simulink model "APP_ChkSig1"  (R2016b)
settings: configuration reference "CodeGenConfigSet" (kept outside this file)
values from neighbouring files (symbols this model uses):
  APP_drLimNeg_C = Calibration.Parameter    [init_APP_ChkSig.m]    (also in init_APP_ChkSig_SIL.m = Simulink.Parameter)
  APP_drLimpMax_C = Calibration.Parameter    [init_APP_ChkSig.m]    (also in init_APP_ChkSig_SIL.m = Simulink.Parameter)
  APP_drLimPos_C = Calibration.Parameter    [init_APP_ChkSig.m]    (also in init_APP_ChkSig_SIL.m = Simulink.Parameter)
  APP_rLimpMax_C = Calibration.Parameter    [init_APP_ChkSig.m]    (also in init_APP_ChkSig_SIL.m = Simulink.Parameter)
  APP_rPlaMaxVal_C = Calibration.Parameter    [init_APP_ChkSig.m]    (also in init_APP_ChkSig_SIL.m = Simulink.Parameter)
  APP_rRmtAPPThresTrqDem_C = Calibration.Parameter    [init_APP_ChkSig.m]    (also in init_APP_ChkSig_SIL.m = Simulink.Parameter)
  APP_rRmtAPPThresTrqDemH_C = Calibration.Parameter    [init_APP_ChkSig.m]    (also in init_APP_ChkSig_SIL.m = Simulink.Parameter)
  APP_rRmtAPPThresTrqDemL_C = Calibration.Parameter    [init_APP_ChkSig.m]    (also in init_APP_ChkSig_SIL.m = Simulink.Parameter)
  APP_rThresAliveDet_C = Calibration.Parameter    [init_APP_ChkSig.m]    (also in init_APP_ChkSig_SIL.m = Simulink.Parameter)
  APP_stRmtAppTrqEN_C = Calibration.Parameter    [init_APP_ChkSig.m]    (also in init_APP_ChkSig_SIL.m = Simulink.Parameter)
  APP_swtAliveDetEna_C = Calibration.Parameter    [init_APP_ChkSig.m]    (also in init_APP_ChkSig_SIL.m = Simulink.Parameter)
  APP_swtPlaChkEna_C = Calibration.Parameter    [init_APP_ChkSig.m]    (also in init_APP_ChkSig_SIL.m = Simulink.Parameter)
  APP_tiAliveDebHiLo_C = Calibration.Parameter    [init_APP_ChkSig.m]    (also in init_APP_ChkSig_SIL.m = Simulink.Parameter)
  APP_tiAliveDebLoHi_C = Calibration.Parameter    [init_APP_ChkSig.m]    (also in init_APP_ChkSig_SIL.m = Simulink.Parameter)
  APP_tiRmtAppEN_C = Calibration.Parameter    [init_APP_ChkSig.m]    (also in init_APP_ChkSig_SIL.m = Simulink.Parameter)
undefined symbols (not defined in the file or in its folder): APP_ChkSig_DT, Switch_conv
libraries: CXLib x11
settings Model: Creator=lenovo  LastModifiedBy=xuxingpei
settings ConfigSetRef: SourceLocation=Base Workspace

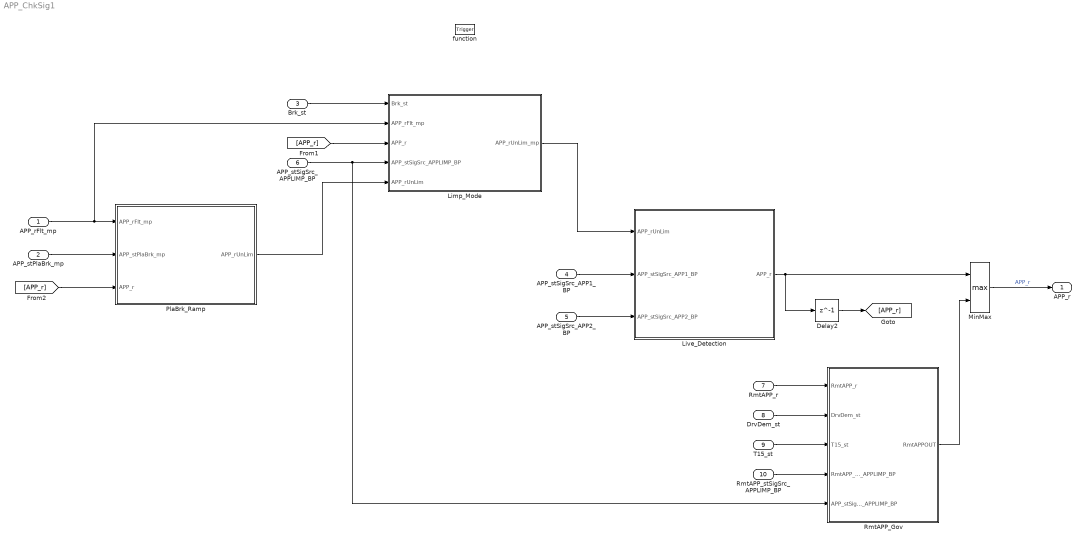
== system APP_ChkSig1 ==
  APP_rFlt_mp : Inport  Tag=%  Description=Acceleration pedal position filtered value  OutMin=0  OutMax=100  OutDataTypeStr=Accpedal_rate
  APP_stPlaBrk_mp : Inport  Description=State of plausibility APP with brake  Port=2  OutMin=0  OutMax=1  OutDataTypeStr=boolean
  Brk_st : Inport  Description=Brake switch state  Port=3  OutMin=0  OutMax=255  OutDataTypeStr=State_uint8
  APP_stSigSrc_APP1_BP : Inport  Description=Sensor 1 is the reference variable, Sensor 2 value is defective  Port=4  OutMin=0  OutMax=1  OutDataTypeStr=boolean
  APP_stSigSrc_APP2_BP : Inport  Description=Sensor 2 is the reference variable,Sensor1 value is defective  Port=5  OutMin=0  OutMax=1  OutDataTypeStr=boolean
  APP_stSigSrc_APPLIMP_BP : Inport  Description=Substitute operation active, accelerator pedal sensor value and accelerator pedal sensor increase are limited  Port=6  OutMin=0  OutMax=1  OutDataTypeStr=boolean
  RmtAPP_r : Inport  Tag=%  Description=Value of Remote accelerator pedal Position  Port=7  OutMin=0  OutMax=100  OutDataTypeStr=Accpedal_rate
  DrvDem_st : Inport  Description=Drive demand status to select the pedal for setpoint calculation  Port=8  OutMin=0  OutMax=255  OutDataTypeStr=State_uint8
  T15_st : Inport  Description=Terminal 15 status after debouncing  Port=9  OutDataTypeStr=Enum: Switch_conv
  RmtAPP_stSigSrc_APPLIMP_BP : Inport  Description=Substitute operation active, remote accelerator pedal sensor value and accelerator pedal sensor increase are limited  Port=10  OutMin=0  OutMax=1  OutDataTypeStr=boolean
  function : TriggerPort  TriggerType=function-call  VariantControl=Variant
  Delay2 : Delay  DelayLength=1  InitialCondition=0
  Limp_Mode : Subsystem
  Live_Detection : Subsystem
  MinMax : MinMax  Function=max  Inputs=2
  PlaBrk_Ramp : Subsystem
  RmtAPP_Gov : Subsystem
  APP_r : Outport  Tag=%  Description=Acceleration pedal sensor 1 value after fault handling  OutMin=0  OutMax=100  OutDataTypeStr=Accpedal_rate
  wires:
  Live_Detection/1(APP_r) -> MinMax/1, Delay2/1
  [APP_r] -> PlaBrk_Ramp/3(APP_r)
  [APP_r] -> Limp_Mode/3(APP_r)
  PlaBrk_Ramp/1(APP_rUnLim) -> Limp_Mode/5(APP_rUnLim)
  Delay2/1 -> [APP_r]
  Limp_Mode/1(APP_rUnLim_mp) -> Live_Detection/1(APP_rUnLim)
  APP_rFlt_mp/1 -> Limp_Mode/2(APP_rFlt_mp), PlaBrk_Ramp/1(APP_rFlt_mp)
  APP_stPlaBrk_mp/1 -> PlaBrk_Ramp/2(APP_stPlaBrk_mp)
  Brk_st/1 -> Limp_Mode/1(Brk_st)
  APP_stSigSrc_APP1_BP/1 -> Live_Detection/2(APP_stSigSrc_APP1_BP)
  APP_stSigSrc_APP2_BP/1 -> Live_Detection/3(APP_stSigSrc_APP2_BP)
  MinMax/1 -> APP_r/1  "APP_r"
  APP_stSigSrc_APPLIMP_BP/1 -> RmtAPP_Gov/5(APP_stSigSrc_APPLIMP_BP), Limp_Mode/4(APP_stSigSrc_APPLIMP_BP)
  RmtAPP_r/1 -> RmtAPP_Gov/1(RmtAPP_r)
  T15_st/1 -> RmtAPP_Gov/3(T15_st)
  DrvDem_st/1 -> RmtAPP_Gov/2(DrvDem_st)
  RmtAPP_Gov/1(RmtAPPOUT) -> MinMax/2
  RmtAPP_stSigSrc_APPLIMP_BP/1 -> RmtAPP_Gov/4(RmtAPP_stSigSrc_APPLIMP_BP)

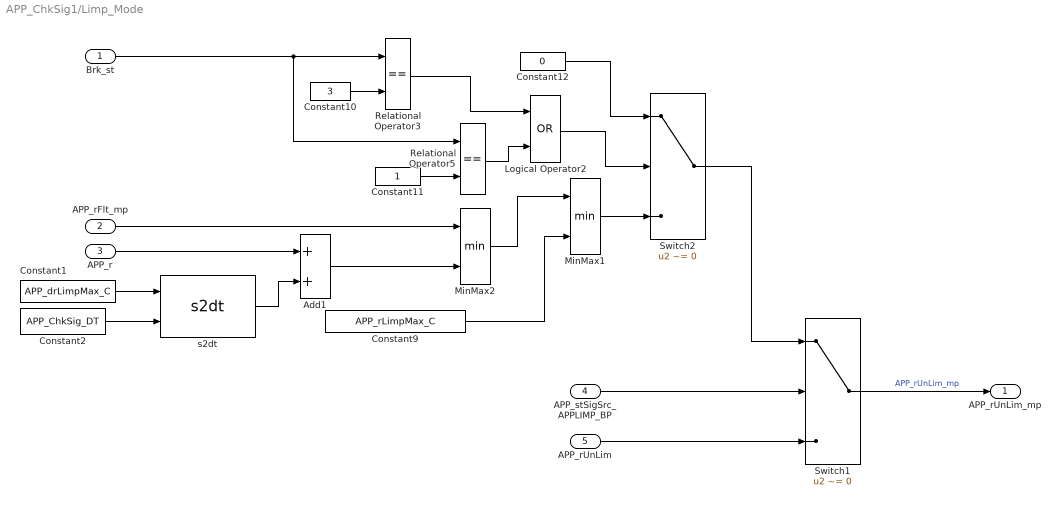
== system APP_ChkSig1/Limp_Mode ==
  Brk_st : Inport
  APP_rFlt_mp : Inport  Port=2
  APP_r : Inport  Port=3
  APP_stSigSrc_APPLIMP_BP : Inport  Tag=-  Description=|  Port=4
      | Substitute operation active, accelerator pedal sensor value and accelerator pedal sensor increase are
      | limited
  APP_rUnLim : Inport  Tag=-  Description=|  Port=5
      | Substitute operation active, accelerator pedal sensor value and accelerator pedal sensor increase are
      | limited
  Add1 : Sum  InputSameDT=on
  Constant1 : Constant  RequirementInfo={'other' 'APP_requirements.doc' '@Simulink_requirement_item_29' 'true' '跛行回家模式' '' } %GIDa_353f93fe_80ad_4b3c_8f6d_af167a07c99e  Value=APP_drLimpMax_C
  Constant10 : Constant  RequirementInfo={'other' 'APP_requirements.doc' '@Simulink_requirement_item_29' 'true' '跛行回家模式' '' } %GIDa_e7d5cc08_b5a3_4c4d_9ed3_8b07ac7e8ac9  Value=3  OutDataTypeStr=Inherit: Inherit via back propagation
  Constant11 : Constant  RequirementInfo={'other' 'APP_requirements.doc' '@Simulink_requirement_item_29' 'true' '跛行回家模式' '' } %GIDa_171f78e0_85dc_4af5_95b3_51a9d06daaa2  OutDataTypeStr=Inherit: Inherit via back propagation
  Constant12 : Constant  RequirementInfo={'other' 'APP_requirements.doc' '@Simulink_requirement_item_29' 'true' '跛行回家模式' '' } %GIDa_1451065e_75e1_4ee1_8d57_18f559653ffb  Value=0  OutDataTypeStr=Inherit: Inherit via back propagation
  Constant2 : Constant  Value=APP_ChkSig_DT  OutDataTypeStr=Inherit: Inherit via back propagation
  Constant9 : Constant  Value=APP_rLimpMax_C
  Logical Operator2 : Logic  RequirementInfo={'other' 'APP_requirements.doc' '@Simulink_requirement_item_29' 'true' '跛行回家模式' '' } %GIDa_91e6f844_91d3_4bd6_ad0e_5784f7c4d80d  Operator=OR  OutDataTypeStr=boolean
  MinMax1 : MinMax  RequirementInfo={'other' 'APP_requirements.doc' '@Simulink_requirement_item_29' 'true' '跛行回家模式' '' } %GIDa_5ea65601_d774_4c9c_9cdf_86ed34ce8d4e  Inputs=2  InputSameDT=on
  MinMax2 : MinMax  RequirementInfo={'other' 'APP_requirements.doc' '@Simulink_requirement_item_29' 'true' '跛行回家模式' '' } %GIDa_09e3386c_7fb5_442c_8bd4_c312d7bcdedf  Inputs=2  InputSameDT=on
  Relational Operator3 : RelationalOperator  RequirementInfo={'other' 'APP_requirements.doc' '@Simulink_requirement_item_29' 'true' '跛行回家模式' '' } %GIDa_9e6d37c3_f581_45ac_9e1d_d077d4155cba  Operator===  OutDataTypeStr=boolean  RndMeth=Nearest  InputSameDT=on
  Relational Operator5 : RelationalOperator  RequirementInfo={'other' 'APP_requirements.doc' '@Simulink_requirement_item_29' 'true' '跛行回家模式' '' } %GIDa_28129197_dd49_49bf_91ce_4055e40024ed  Operator===  OutDataTypeStr=boolean  RndMeth=Nearest  InputSameDT=on
  Switch1 : Switch  RequirementInfo={'other' 'APP_requirements.doc' '@Simulink_requirement_item_29' 'true' '跛行回家模式' '' } %GIDa_2ac1c5af_0938_42ef_9cc7_76d7410514c3  Criteria=u2 ~= 0
  Switch2 : Switch  RequirementInfo={'other' 'APP_requirements.doc' '@Simulink_requirement_item_29' 'true' '跛行回家模式' '' } %GIDa_af6b6881_5585_4ba9_a6b7_f15e855fb530  Criteria=u2 ~= 0  InputSameDT=on
  s2dt : CXLib/s2dt
  APP_rUnLim_mp : Outport
  wires:
  APP_rFlt_mp/1 -> MinMax2/1
  Constant10/1 -> Relational Operator3/2
  Switch2/1 -> Switch1/1
  Brk_st/1 -> Relational Operator3/1, Relational Operator5/1
  Relational Operator3/1 -> Logical Operator2/1
  Constant11/1 -> Relational Operator5/2
  Constant9/1 -> MinMax1/2
  APP_r/1 -> Add1/1
  MinMax2/1 -> MinMax1/1
  Add1/1 -> MinMax2/2
  MinMax1/1 -> Switch2/3
  Logical Operator2/1 -> Switch2/2
  Constant12/1 -> Switch2/1
  Relational Operator5/1 -> Logical Operator2/2
  APP_rUnLim/1 -> Switch1/3
  APP_stSigSrc_APPLIMP_BP/1 -> Switch1/2
  Switch1/1 -> APP_rUnLim_mp/1  "APP_rUnLim_mp"
  Constant1/1 -> s2dt/1
  s2dt/1 -> Add1/2
  Constant2/1 -> s2dt/2

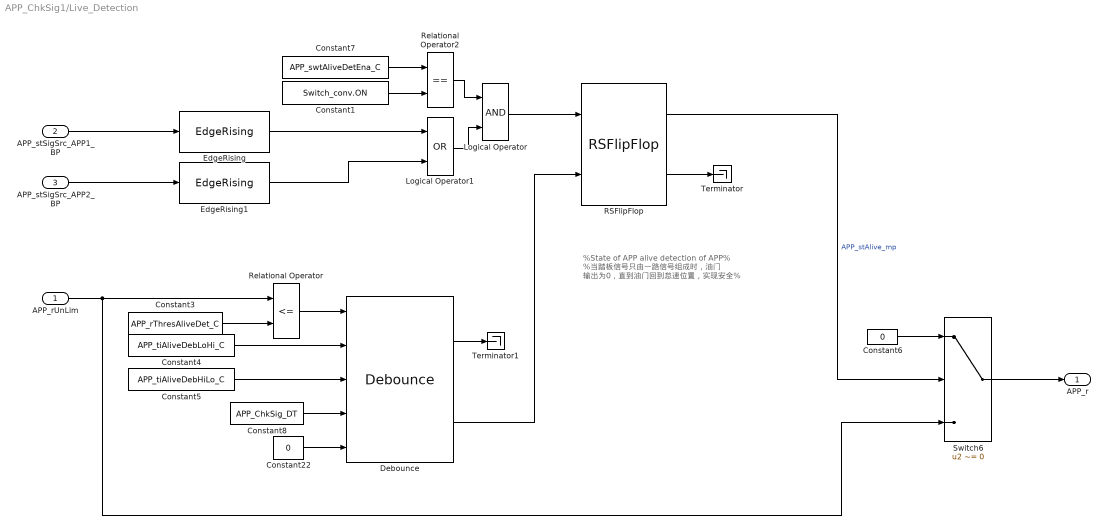
== system APP_ChkSig1/Live_Detection ==
  note: %State of APP alive detection of APP%
      | %当踏板信号只由一路信号组成时，油门
      | 输出为0，直到油门回到怠速位置，实现安全%
  APP_rUnLim : Inport
  APP_stSigSrc_APP1_BP : Inport  Port=2
  APP_stSigSrc_APP2_BP : Inport  Port=3
  Constant1 : Constant  RequirementInfo={'other' 'APP_requirements.doc' '@Simulink_requirement_item_28' 'true' '油门保护模式' '' } %GIDa_36ea5633_4c55_4f8a_bf6e_0a140dfab8df  Value=Switch_conv.ON  OutDataTypeStr=Inherit: Inherit via back propagation
  Constant22 : Constant  Value=0  OutDataTypeStr=Inherit: Inherit via back propagation
  Constant3 : Constant  RequirementInfo={'other' 'APP_requirements.doc' '@Simulink_requirement_item_28' 'true' '油门保护模式' '' } %GIDa_0f293ffd_d384_4524_9e66_a89ae430d534  Value=APP_rThresAliveDet_C
  Constant4 : Constant  Value=APP_tiAliveDebLoHi_C
  Constant5 : Constant  Value=APP_tiAliveDebHiLo_C
  Constant6 : Constant  Value=0  OutDataTypeStr=Inherit: Inherit via back propagation
  Constant7 : Constant  RequirementInfo={'other' 'APP_requirements.doc' '@Simulink_requirement_item_28' 'true' '油门保护模式' '' } %GIDa_c046e833_1f46_4c1b_95a2_918fd5382666  Value=APP_swtAliveDetEna_C
  Constant8 : Constant  Value=APP_ChkSig_DT  OutDataTypeStr=Inherit: Inherit via back propagation
  Debounce : CXLib/Debounce  RequirementInfo={'other' 'APP_requirements.doc' '@Simulink_requirement_item_28' 'true' '油门保护模式' '' } %GIDa_968da003_69be_421b_938d_9c0798a98bce
  EdgeRising : CXLib/EdgeRising
  EdgeRising1 : CXLib/EdgeRising
  Logical Operator : Logic  OutDataTypeStr=boolean
  Logical Operator1 : Logic  Operator=OR  OutDataTypeStr=boolean
  RSFlipFlop : CXLib/RSFlipFlop
  Relational Operator : RelationalOperator  RequirementInfo={'other' 'APP_requirements.doc' '@Simulink_requirement_item_28' 'true' '油门保护模式' '' } %GIDa_aeb668a3_40d5_4fbf_8422_c8e18de92290  Operator=<=  OutDataTypeStr=boolean  RndMeth=Nearest  InputSameDT=on
  Relational Operator2 : RelationalOperator  RequirementInfo={'other' 'APP_requirements.doc' '@Simulink_requirement_item_28' 'true' '油门保护模式' '' } %GIDa_d45ec2eb_89c7_4ded_aad0_d6882c77a116  Operator===  OutDataTypeStr=boolean  RndMeth=Nearest  InputSameDT=on
  Switch6 : Switch  Criteria=u2 ~= 0  InputSameDT=on
  Terminator : Terminator
  Terminator1 : Terminator
  APP_r : Outport
  wires:
  Debounce/1 -> Terminator1/1
  Constant22/1 -> Debounce/5
  Logical Operator/1 -> RSFlipFlop/1
  RSFlipFlop/2 -> Terminator/1
  Logical Operator1/1 -> Logical Operator/2
  Relational Operator/1 -> Debounce/1
  APP_stSigSrc_APP1_BP/1 -> EdgeRising/1
  Debounce/2 -> RSFlipFlop/2
  Constant1/1 -> Relational Operator2/2
  Constant7/1 -> Relational Operator2/1
  Relational Operator2/1 -> Logical Operator/1
  RSFlipFlop/1 -> Switch6/2  "APP_stAlive_mp"
  Constant5/1 -> Debounce/3
  Constant4/1 -> Debounce/2
  Constant3/1 -> Relational Operator/2
  Constant8/1 -> Debounce/4
  APP_rUnLim/1 -> Switch6/3, Relational Operator/1
  Constant6/1 -> Switch6/1
  EdgeRising/1 -> Logical Operator1/1
  APP_stSigSrc_APP2_BP/1 -> EdgeRising1/1
  EdgeRising1/1 -> Logical Operator1/2
  Switch6/1 -> APP_r/1

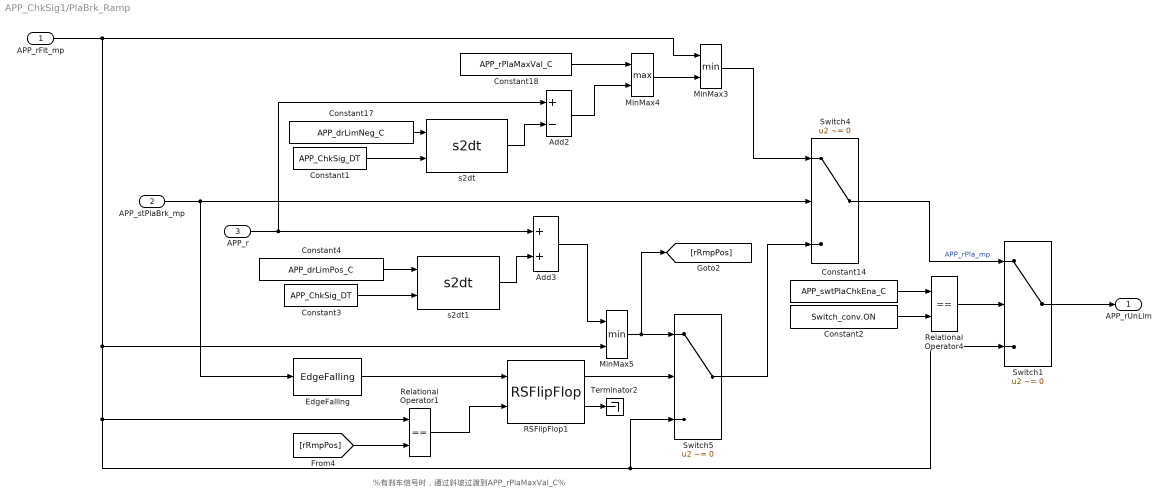
== system APP_ChkSig1/PlaBrk_Ramp ==
  note: %有刹车信号时，通过斜坡过渡到APP_rPlaMaxVal_C%
  APP_rFlt_mp : Inport  RequirementInfo={'other' 'APP_requirements.doc' '@Simulink_requirement_item_30' 'true' '刹车故障模式' '' } %GIDa_4fe30265_16ee_4199_92b3_9e13d7110139
  APP_stPlaBrk_mp : Inport  RequirementInfo={'other' 'APP_requirements.doc' '@Simulink_requirement_item_30' 'true' '刹车故障模式' '' } %GIDa_7110d923_40c0_441b_94ea_fe486c0b454d  Port=2
  APP_r : Inport  RequirementInfo={'other' 'APP_requirements.doc' '@Simulink_requirement_item_30' 'true' '刹车故障模式' '' } %GIDa_427cec16_09ac_4e1a_b543_dca640d6b0d6  Port=3
  Add2 : Sum  Inputs=+-  InputSameDT=on
  Add3 : Sum  InputSameDT=on
  Constant1 : Constant  Value=APP_ChkSig_DT  OutDataTypeStr=Inherit: Inherit via back propagation
  Constant14 : Constant  RequirementInfo={'other' 'APP_requirements.doc' '@Simulink_requirement_item_30' 'true' '刹车故障模式' '' } %GIDa_ea8af942_b90f_49c1_ae44_70d8690d4b00  Value=APP_swtPlaChkEna_C
  Constant17 : Constant  Value=APP_drLimNeg_C
  Constant18 : Constant  RequirementInfo={'other' 'APP_requirements.doc' '@Simulink_requirement_item_30' 'true' '刹车故障模式' '' } %GIDa_815fef24_eef6_4ba8_b25d_c30568dc96af  Value=APP_rPlaMaxVal_C
  Constant2 : Constant  RequirementInfo={'other' 'APP_requirements.doc' '@Simulink_requirement_item_28' 'true' '油门保护模式' '' } %GIDa_cad408c8_2bed_48e1_96bd_7b693d634e62  Value=Switch_conv.ON  OutDataTypeStr=Inherit: Inherit via back propagation
  Constant3 : Constant  Value=APP_ChkSig_DT  OutDataTypeStr=Inherit: Inherit via back propagation
  Constant4 : Constant  Value=APP_drLimPos_C
  EdgeFalling : CXLib/EdgeFalling
  MinMax3 : MinMax  Inputs=2  InputSameDT=on
  MinMax4 : MinMax  Function=max  Inputs=2  InputSameDT=on
  MinMax5 : MinMax  Inputs=2  InputSameDT=on
  RSFlipFlop1 : CXLib/RSFlipFlop
  Relational Operator1 : RelationalOperator  RequirementInfo={'other' 'APP_requirements.doc' '@Simulink_requirement_item_29' 'true' '跛行回家模式' '' } %GIDa_7c4cc187_faf4_4e6c_8787_c34c8ec11c45  Operator===  OutDataTypeStr=boolean  RndMeth=Nearest  InputSameDT=on
  Relational Operator4 : RelationalOperator  RequirementInfo={'other' 'APP_requirements.doc' '@Simulink_requirement_item_28' 'true' '油门保护模式' '' } %GIDa_b0a730e5_b985_4906_a9a7_7ff7fbf896c7  Operator===  OutDataTypeStr=boolean  RndMeth=Nearest  InputSameDT=on
  Switch1 : Switch  RequirementInfo={'other' 'APP_requirements.doc' '@Simulink_requirement_item_30' 'true' '刹车故障模式' '' } %GIDa_5e1a9e03_d48a_4c7e_9b24_9896d8e0ff8c  Criteria=u2 ~= 0  OutDataTypeStr=Inherit: Inherit via back propagation
  Switch4 : Switch  RequirementInfo={'other' 'APP_requirements.doc' '@Simulink_requirement_item_30' 'true' '刹车故障模式' '' } %GIDa_57635b49_58cf_4091_8abb_96acf666cbc4  Criteria=u2 ~= 0  InputSameDT=on
  Switch5 : Switch  RequirementInfo={'other' 'APP_requirements.doc' '@Simulink_requirement_item_30' 'true' '刹车故障模式' '' } %GIDa_4104dd93_6342_4756_9b78_8955c31e288d  Criteria=u2 ~= 0  InputSameDT=on
  Terminator2 : Terminator
  s2dt : CXLib/s2dt
  s2dt1 : CXLib/s2dt
  APP_rUnLim : Outport
  wires:
  APP_rFlt_mp/1 -> MinMax3/1, Switch5/3, Switch1/3, Relational Operator1/1, MinMax5/2
  s2dt1/1 -> Add3/2
  EdgeFalling/1 -> RSFlipFlop1/1
  Relational Operator1/1 -> RSFlipFlop1/2
  [rRmpPos] -> Relational Operator1/2
  Add2/1 -> MinMax4/2
  APP_r/1 -> Add3/1, Add2/1
  Relational Operator4/1 -> Switch1/2
  RSFlipFlop1/2 -> Terminator2/1
  Constant2/1 -> Relational Operator4/2
  Switch5/1 -> Switch4/3
  Constant18/1 -> MinMax4/1
  MinMax4/1 -> MinMax3/2
  Switch4/1 -> Switch1/1  "APP_rPla_mp"
  Add3/1 -> MinMax5/1
  MinMax5/1 -> [rRmpPos], Switch5/1
  RSFlipFlop1/1 -> Switch5/2
  APP_stPlaBrk_mp/1 -> Switch4/2, EdgeFalling/1
  Switch1/1 -> APP_rUnLim/1
  MinMax3/1 -> Switch4/1
  Constant14/1 -> Relational Operator4/1
  Constant1/1 -> s2dt/2
  Constant17/1 -> s2dt/1
  s2dt/1 -> Add2/2
  Constant3/1 -> s2dt1/2
  Constant4/1 -> s2dt1/1

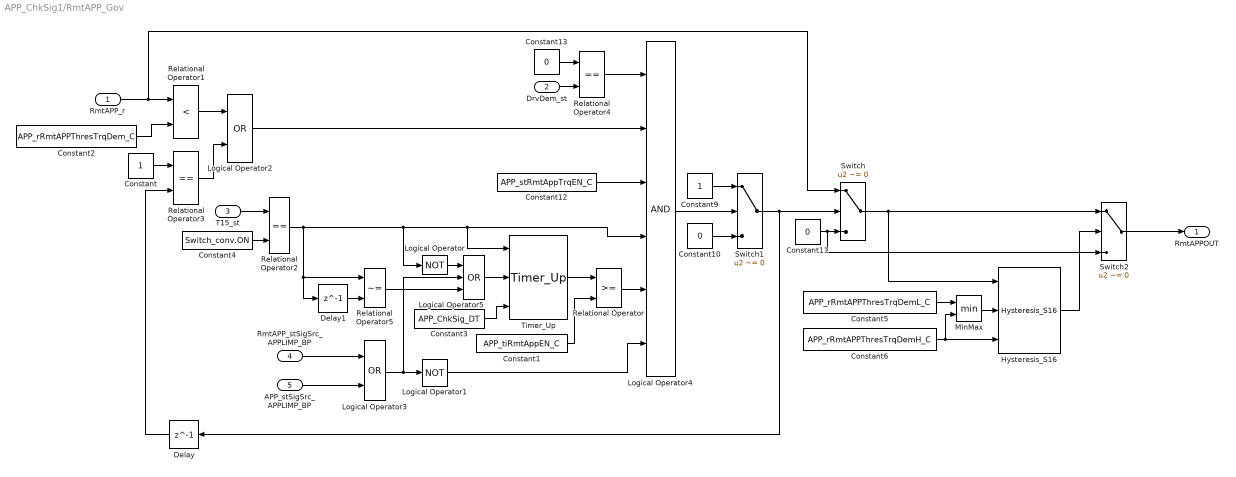
== system APP_ChkSig1/RmtAPP_Gov ==
  RmtAPP_r : Inport  Tag=%  Description=Value of Remote accelerator pedal Position  OutMin=0  OutMax=100  OutDataTypeStr=Accpedal_rate
  DrvDem_st : Inport  Port=2
  T15_st : Inport  Port=3
  RmtAPP_stSigSrc_APPLIMP_BP : Inport  Port=4
  APP_stSigSrc_APPLIMP_BP : Inport  Description=Substitute operation active, accelerator pedal sensor value and accelerator pedal sensor increase are limited  Port=5  OutMin=0  OutMax=1  OutDataTypeStr=boolean
  Constant : Constant  OutDataTypeStr=Inherit: Inherit via back propagation
  Constant1 : Constant  Value=APP_tiRmtAppEN_C
  Constant10 : Constant  Value=0  OutDataTypeStr=boolean
  Constant11 : Constant  Value=0  OutDataTypeStr=Inherit: Inherit via back propagation
  Constant12 : Constant  Value=APP_stRmtAppTrqEN_C
  Constant13 : Constant  Value=0  OutDataTypeStr=Inherit: Inherit via back propagation
  Constant2 : Constant  Value=APP_rRmtAPPThresTrqDem_C
  Constant3 : Constant  Value=APP_ChkSig_DT
  Constant4 : Constant  Value=Switch_conv.ON
  Constant5 : Constant  Value=APP_rRmtAPPThresTrqDemL_C
  Constant6 : Constant  Value=APP_rRmtAPPThresTrqDemH_C
  Constant9 : Constant  OutDataTypeStr=Inherit: Inherit via back propagation
  Delay : Delay  DelayLength=1  InitialCondition=0
  Delay1 : Delay  DelayLength=1  InitialCondition=0
  Hysteresis_S16 : CXLib/Hysteresis_S16
  Logical Operator : Logic  Operator=NOT  AllPortsSameDT=off  OutDataTypeStr=boolean
  Logical Operator1 : Logic  Operator=NOT  AllPortsSameDT=off  OutDataTypeStr=boolean
  Logical Operator2 : Logic  Operator=OR  OutDataTypeStr=boolean
  Logical Operator3 : Logic  Operator=OR  AllPortsSameDT=off  OutDataTypeStr=boolean
  Logical Operator4 : Logic  Inputs=6  AllPortsSameDT=off  OutDataTypeStr=boolean
  Logical Operator5 : Logic  Operator=OR  Inputs=3  AllPortsSameDT=off  OutDataTypeStr=boolean
  MinMax : MinMax  Inputs=2
  Relational Operator : RelationalOperator  OutDataTypeStr=boolean  RndMeth=Simplest
  Relational Operator1 : RelationalOperator  Operator=<  OutDataTypeStr=boolean  RndMeth=Nearest  InputSameDT=on
  Relational Operator2 : RelationalOperator  Operator===  OutDataTypeStr=boolean  RndMeth=Simplest
  Relational Operator3 : RelationalOperator  Operator===  OutDataTypeStr=boolean  RndMeth=Nearest  InputSameDT=on
  Relational Operator4 : RelationalOperator  Operator===  OutDataTypeStr=boolean  RndMeth=Simplest  InputSameDT=on
  Relational Operator5 : RelationalOperator  Operator=~=  OutDataTypeStr=boolean  RndMeth=Simplest
  Switch : Switch  Criteria=u2 ~= 0
  Switch1 : Switch  Criteria=u2 ~= 0
  Switch2 : Switch  Criteria=u2 ~= 0
  Timer_Up : CXLib/Timer_Up
  RmtAPPOUT : Outport
  wires:
  Constant2/1 -> Relational Operator1/2
  Delay/1 -> Relational Operator3/2
  Constant/1 -> Relational Operator3/1
  Switch1/1 -> Switch/2, Delay/1
  Constant11/1 -> Switch2/3, Switch/3
  DrvDem_st/1 -> Relational Operator4/2
  Relational Operator1/1 -> Logical Operator2/1
  Constant9/1 -> Switch1/1
  RmtAPP_r/1 -> Switch/1, Relational Operator1/1
  Relational Operator3/1 -> Logical Operator2/2
  Logical Operator4/1 -> Switch1/2
  Constant10/1 -> Switch1/3
  Constant13/1 -> Relational Operator4/1
  Logical Operator2/1 -> Logical Operator4/2
  Constant12/1 -> Logical Operator4/3
  Relational Operator4/1 -> Logical Operator4/1
  T15_st/1 -> Relational Operator2/1
  Timer_Up/1 -> Relational Operator/1
  Constant1/1 -> Relational Operator/2
  Constant3/1 -> Timer_Up/3
  Relational Operator/1 -> Logical Operator4/5
  Logical Operator1/1 -> Logical Operator4/6
  APP_stSigSrc_APPLIMP_BP/1 -> Logical Operator3/2
  Logical Operator3/1 -> Logical Operator1/1, Logical Operator5/2
  RmtAPP_stSigSrc_APPLIMP_BP/1 -> Logical Operator3/1
  Logical Operator5/1 -> Timer_Up/2
  Logical Operator/1 -> Logical Operator5/1
  Constant4/1 -> Relational Operator2/2
  Delay1/1 -> Relational Operator5/2
  Relational Operator5/1 -> Logical Operator5/3
  Relational Operator2/1 -> Logical Operator/1, Logical Operator4/4, Timer_Up/1, Delay1/1, Relational Operator5/1
  Switch/1 -> Switch2/1, Hysteresis_S16/1
  Constant6/1 -> MinMax/2, Hysteresis_S16/3
  Hysteresis_S16/1 -> Switch2/2
  Switch2/1 -> RmtAPPOUT/1
  MinMax/1 -> Hysteresis_S16/2
  Constant5/1 -> MinMax/1
